simulink library "lib_finite_difference_derivative"  (R2023a)
settings: Solver=VariableStepAuto  StartTime=0.0  StopTime=10.0  RelTol=1e-3
libraries: lib_conversion x4
settings Model: Creator=RAN2OFO  LastModifiedBy=lenovo
settings OptimizationCC: ReuseModelBlockBuffer=off

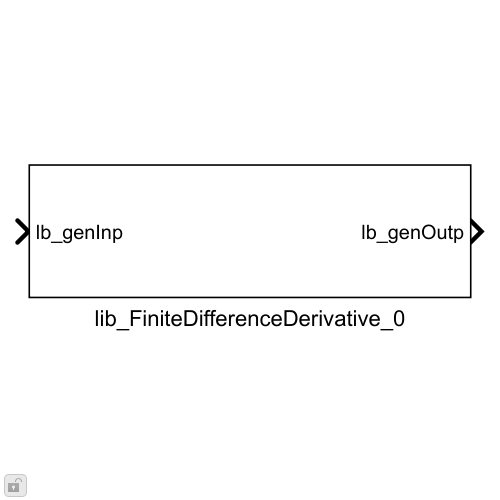
[thumbnail: Simulink's stored preview of the top-level diagram]
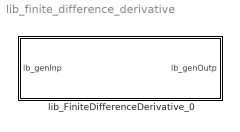
== system lib_finite_difference_derivative ==
  lib_FiniteDifferenceDerivative_0 : Subsystem  mask{lb_parSampTime=0.01, lb_parMaxInpVar=0.1, lb_parOutpPhyPek=4096, lb_parAngInpMode=on, lb_parOutpDataType=fixdt(1,16,2^0,0)}
      mask prompts: lb_parSampTime "Sampling time [s]:"; lb_parMaxInpVar "Maximum input variation (u(k)-u(k-1)):"; lb_parOutpPhyPek "Peak output physical value:"; lb_parAngInpMode "Angle input mode"; lb_parOutpDataType "Output data type:"
      mask init:
      | parMaxInpVar = double(lb_parMaxInpVar);
      | parSampTime = double(lb_parSampTime);
      | 
      | if lb_parAngInpMode
      |     set_param([gcb,'/vss_AngleModeSelection'],'LabelModeActiveChoice','lb_parAngInpModeLbl');
      | else
      |     set_param([gcb,'/vss_AngleModeSelection'],'LabelModeActiveChoice','lb_parGenInpModeLbl');
      | end
      | 
      | %% Req. XXX_ Define data type for product (u-u_pre)*cf
      | lb_parDevMaxVal = parMaxInpVar/parSampTime;
      | lb_parDevDataType = Simulink.NumericType;
      | lb_parDevDataType.DataTypeMode= 'Fixed-point: unspecified scaling';
      | lb_parDevDataType.Signedness = 'Signed';
      | lb_parDevDataType.WordLength = 16;
      mask DialogControl DescGroupVar Prompt: WeiFu control Library
      mask DialogControl DescTextVar Prompt: Finite difference derivative block
      mask DialogControl parDesc Prompt: Parameters
      mask DialogControl Container4 Prompt: Operating mode
      mask DialogControl dataTypeDesc Prompt: Data type

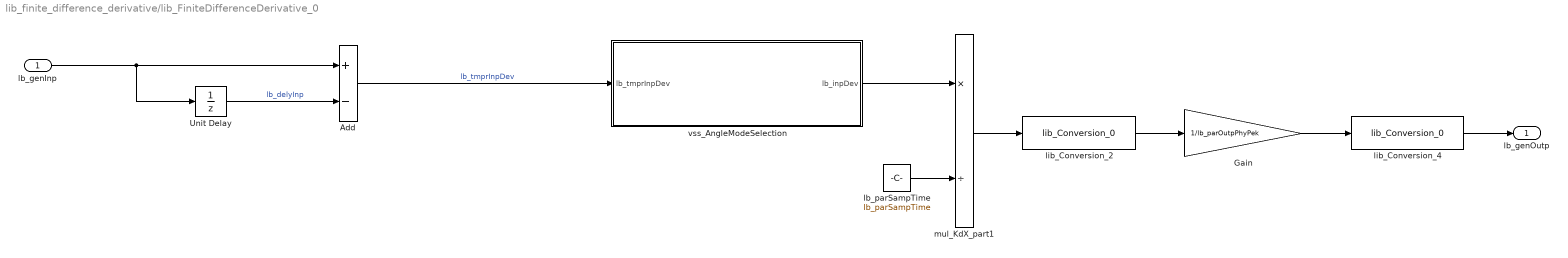
== system lib_finite_difference_derivative/lib_FiniteDifferenceDerivative_0 ==
  lb_genInp : Inport
  Add : Sum  Inputs=+-  OutDataTypeStr=Inherit: Inherit via back propagation  RndMeth=Simplest
  Gain : Gain  Gain=1/lb_parOutpPhyPek  OutDataTypeStr=Inherit: Inherit via back propagation
  Unit Delay : UnitDelay  SampleTime=-1  HasFrameUpgradeWarning=on
  lb_parSampTime : Constant  Value=lb_parSampTime
  lib_Conversion_2 : lib_conversion/lib_Conversion_0  lb_parDataType=lb_parDevDataType  lb_parOutpMaxVal=lb_parDevMaxVal  lb_parOutpMinVal=[]  lb_parSatFlag=off
  lib_Conversion_4 : lib_conversion/lib_Conversion_0  lb_parDataType=lb_parOutpDataType  lb_parOutpMaxVal=[]  lb_parOutpMinVal=[]  lb_parSatFlag=off
  mul_KdX_part1 : Product  Inputs=*/  OutDataTypeStr=Inherit: Inherit via back propagation  RndMeth=Simplest
  vss_AngleModeSelection : Subsystem  Variant=on  VariantControlMode=label  LabelModeActiveChoice=lb_parAngInpModeLbl
  lb_genOutp : Outport
  wires:
  lib_Conversion_4/1 -> lb_genOutp/1
  lb_parSampTime/1 -> mul_KdX_part1/2
  lb_genInp/1 -> Add/1, Unit Delay/1
  Unit Delay/1 -> Add/2  "lb_delyInp"
  Add/1 -> vss_AngleModeSelection/1(lb_tmprInpDev)  "lb_tmprInpDev"
  Gain/1 -> lib_Conversion_4/1
  mul_KdX_part1/1 -> lib_Conversion_2/1
  vss_AngleModeSelection/1(lb_inpDev) -> mul_KdX_part1/1
  lib_Conversion_2/1 -> Gain/1

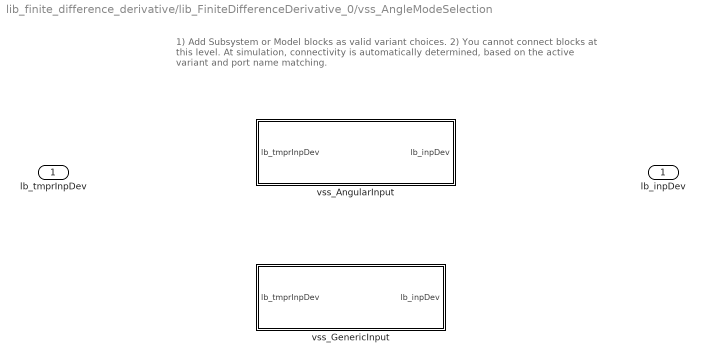
== system lib_finite_difference_derivative/lib_FiniteDifferenceDerivative_0/vss_AngleModeSelection ==
  note: 1) Add Subsystem or Model blocks as valid variant choices.
      | 2) You cannot connect blocks at this level. At simulation, connectivity is automatically
      | determined, based on the active variant and port name matching.
  lb_tmprInpDev : Inport
  vss_AngularInput : Subsystem  VariantControl=lb_parAngInpModeLbl
  vss_GenericInput : Subsystem  VariantControl=lb_parGenInpModeLbl
  lb_inpDev : Outport

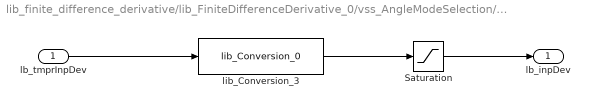
== system lib_finite_difference_derivative/lib_FiniteDifferenceDerivative_0/vss_AngleModeSelection/vss_AngularInput ==
  lb_tmprInpDev : Inport
  Saturation : Saturate  UpperLimit=lb_parMaxInpVar  LowerLimit=-lb_parMaxInpVar
  lib_Conversion_3 : lib_conversion/lib_Conversion_0  lb_parDataType=fixdt(1,16,pi*2^-15,0)  lb_parOutpMaxVal=[]  lb_parOutpMinVal=[]  lb_parSatFlag=off
  lb_inpDev : Outport
  wires:
  lb_tmprInpDev/1 -> lib_Conversion_3/1
  Saturation/1 -> lb_inpDev/1
  lib_Conversion_3/1 -> Saturation/1

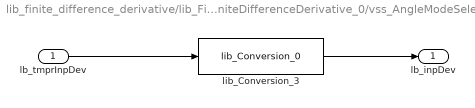
== system lib_finite_difference_derivative/lib_FiniteDifferenceDerivative_0/vss_AngleModeSelection/vss_GenericInput ==
  lb_tmprInpDev : Inport
  lib_Conversion_3 : lib_conversion/lib_Conversion_0  lb_parDataType=fixdt(1,16)  lb_parOutpMaxVal=lb_parMaxInpVar  lb_parOutpMinVal=[]  lb_parSatFlag=off
  lb_inpDev : Outport
  wires:
  lib_Conversion_3/1 -> lb_inpDev/1
  lb_tmprInpDev/1 -> lib_Conversion_3/1
